simulink model "ihc_lowpass_filter"  (R2020b)
settings: Solver=FixedStepDiscrete  StartTime=0.0  StopTime=stopTime  FixedStep=2.0833333333333333e-05  RelTol=1e-3
values from neighbouring files (symbols this model uses):
  IHCLPcoeffs = [ gainihc*c2LPihc gainihc*c2LPihc 0 1 -c1LPihc 0 ... (first row only)    [ihc_lowpass_filter_parameters.m]
settings Model: Creator=Ross  LastModifiedBy=conno
settings DataIOCC: SaveOutput=off  SaveTime=off  ReturnWorkspaceOutputs=off
settings OptimizationCC: BlockReduction=off  ConditionallyExecuteInputs=off  DefaultParameterBehavior=Inlined
settings DebuggingCC: ReadBeforeWriteMsg=DisableAll  WriteAfterWriteMsg=DisableAll  WriteAfterReadMsg=DisableAll  AlgebraicLoopMsg=error  MultiTaskDSMMsg=none  SingleTaskRateTransMsg=error  PregeneratedLibrarySubsystemCodeDiagnostic=none  ArithmeticOperatorsInVariantConditions=warning
settings HardwareCC: ProdBitPerPointer=32  ProdBitPerSizeT=32  ProdBitPerPtrDiffT=32  ProdLargestAtomicFloat=None  ProdIntDivRoundTo=Undefined  ProdEndianess=Unspecified  ProdWordSize=32  ProdHWDeviceType=ASIC/FPGA->ASIC/FPGA  TargetBitPerPointer=64  TargetBitPerSizeT=64  TargetBitPerPtrDiffT=64  TargetLongLongMode=on  TargetIntDivRoundTo=Zero  TargetEndianess=LittleEndian  TargetWordSize=64  TargetHWDeviceType=Custom Processor->MATLAB Host Computer  ProdEqTarget=off
settings ModelReferenceCC: UpdateModelReferenceTargets=IfOutOfDate
settings SFSimCC: SFSimEcho=off  SimUseLocalCustomCode=off  CustomCodeUndefinedFunction=UseInterfaceOnly
settings RTWCC: RTWUseLocalCustomCode=off

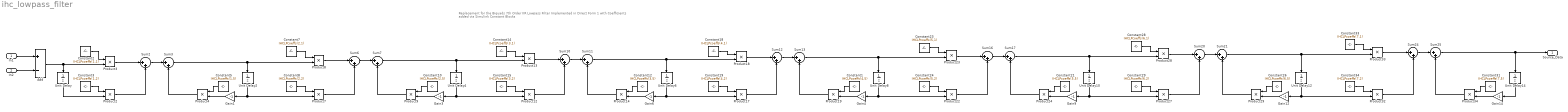
== system ihc_lowpass_filter ==
  note: Replacement for the Biquads
      | 7th Order IIR Lowpass Filter Implemented in Direct Form 1 with Coefficients added via Simulink Constant Blocks
  In1 : Inport  OutDataTypeStr=single  PortDimensions=1  SampleTime=[2.0833333333333333e-05,0]
  In2 : Inport  Port=2  OutDataTypeStr=single  PortDimensions=1  SampleTime=[2.0833333333333333e-05,0]
  Add : Sum  Inputs=+-  RndMeth=Nearest
  Constant1 : Constant  Value=IHCLPcoeffs(4,5)  OutDataTypeStr=single  SampleTime=-1
  Constant10 : Constant  Value=IHCLPcoeffs(2,5)  OutDataTypeStr=single  SampleTime=-1
  Constant12 : Constant  Value=IHCLPcoeffs(3,5)  OutDataTypeStr=single  SampleTime=-1
  Constant14 : Constant  Value=IHCLPcoeffs(3,1)  OutDataTypeStr=single  SampleTime=-1
  Constant15 : Constant  Value=IHCLPcoeffs(3,2)  OutDataTypeStr=single  SampleTime=-1
  Constant18 : Constant  Value=IHCLPcoeffs(4,1)  OutDataTypeStr=single  SampleTime=-1
  Constant19 : Constant  Value=IHCLPcoeffs(4,2)  OutDataTypeStr=single  SampleTime=-1
  Constant2 : Constant  Value=IHCLPcoeffs(1,1)  OutDataTypeStr=single  SampleTime=-1
  Constant21 : Constant  Value=IHCLPcoeffs(5,5)  OutDataTypeStr=single  SampleTime=-1
  Constant23 : Constant  Value=IHCLPcoeffs(5,1)  OutDataTypeStr=single  SampleTime=-1
  Constant24 : Constant  Value=IHCLPcoeffs(5,2)  OutDataTypeStr=single  SampleTime=-1
  Constant26 : Constant  Value=IHCLPcoeffs(6,5)  OutDataTypeStr=single  SampleTime=-1
  Constant28 : Constant  Value=IHCLPcoeffs(6,1)  OutDataTypeStr=single  SampleTime=-1
  Constant29 : Constant  Value=IHCLPcoeffs(6,2)  OutDataTypeStr=single  SampleTime=-1
  Constant3 : Constant  Value=IHCLPcoeffs(1,2)  OutDataTypeStr=single  SampleTime=-1
  Constant31 : Constant  Value=IHCLPcoeffs(7,5)  OutDataTypeStr=single  SampleTime=-1
  Constant33 : Constant  Value=IHCLPcoeffs(7,1)  OutDataTypeStr=single  SampleTime=-1
  Constant34 : Constant  Value=IHCLPcoeffs(7,2)  OutDataTypeStr=single  SampleTime=-1
  Constant5 : Constant  Value=IHCLPcoeffs(1,5)  OutDataTypeStr=single  SampleTime=-1
  Constant7 : Constant  Value=IHCLPcoeffs(2,1)  OutDataTypeStr=single  SampleTime=-1
  Constant8 : Constant  Value=IHCLPcoeffs(2,2)  OutDataTypeStr=single  SampleTime=-1
  Gain{1,3..4,6,9,12,14} (7 alike) : Gain  Gain=-1
  Product{2..4,7..9,12..14,17..19,22..24,27..29,32..34} (21 alike) : Product
  Sum{2..3,6..7,10..13,16..17,20..21,24..25} (14 alike) : Sum  Inputs=|++
  Unit Delay{,2,4,6,8,10,12,14} (8 alike) : UnitDelay  SampleTime=-1  HasFrameUpgradeWarning=on
  Source_Data : Outport  OutDataTypeStr=single  PortDimensions=1  SampleTime=[2.0833333333333333e-05,0]
  wires:
  Constant31/1 -> Product34/1
  Product34/1 -> Sum25/2
  Sum24/1 -> Sum25/1
  Gain14/1 -> Product34/2
  Sum25/1 -> Source_Data/1, Unit Delay14/1
  Product32/1 -> Sum24/2
  Product33/1 -> Sum24/1
  Unit Delay14/1 -> Gain14/1
  Constant34/1 -> Product32/1
  Constant33/1 -> Product33/1
  Constant26/1 -> Product29/1
  Product29/1 -> Sum21/2
  Sum20/1 -> Sum21/1
  Gain12/1 -> Product29/2
  Sum21/1 -> Unit Delay12/1, Product33/2
  Product27/1 -> Sum20/2
  Product28/1 -> Sum20/1
  Unit Delay12/1 -> Product32/2, Gain12/1
  Constant29/1 -> Product27/1
  Constant28/1 -> Product28/1
  Sum12/1 -> Sum13/1
  Constant23/1 -> Product23/1
  Constant2/1 -> Product3/1
  Constant7/1 -> Product8/1
  Add/1 -> Product3/2, Unit Delay/1
  Product8/1 -> Sum6/1
  Constant1/1 -> Product19/1
  Unit Delay4/1 -> Product12/2, Gain3/1
  Product24/1 -> Sum17/2
  Constant24/1 -> Product22/1
  Gain6/1 -> Product14/2
  Sum13/1 -> Unit Delay8/1, Product23/2
  Sum7/1 -> Unit Delay4/1, Product13/2
  Product12/1 -> Sum10/2
  Gain1/1 -> Product4/2
  Product14/1 -> Sum11/2
  Gain4/1 -> Product19/2
  Sum10/1 -> Sum11/1
  Gain9/1 -> Product24/2
  Unit Delay10/1 -> Product27/2, Gain9/1
  Unit Delay6/1 -> Product17/2, Gain6/1
  Product4/1 -> Sum3/2
  Sum11/1 -> Unit Delay6/1, Product18/2
  Product18/1 -> Sum12/1
  Constant15/1 -> Product12/1
  Sum16/1 -> Sum17/1
  Constant19/1 -> Product17/1
  Unit Delay2/1 -> Product7/2, Gain1/1
  Constant21/1 -> Product24/1
  Constant3/1 -> Product2/1
  Product3/1 -> Sum2/1
  Product23/1 -> Sum16/1
  Sum3/1 -> Unit Delay2/1, Product8/2
  Product22/1 -> Sum16/2
  Unit Delay8/1 -> Product22/2, Gain4/1
  Unit Delay/1 -> Product2/2
  Gain3/1 -> Product9/2
  Product17/1 -> Sum12/2
  Product13/1 -> Sum10/1
  Sum17/1 -> Unit Delay10/1, Product28/2
  Constant14/1 -> Product13/1
  Constant12/1 -> Product14/1
  Constant18/1 -> Product18/1
  Product9/1 -> Sum7/2
  Constant5/1 -> Product4/1
  Constant10/1 -> Product9/1
  Product19/1 -> Sum13/2
  Constant8/1 -> Product7/1
  Sum2/1 -> Sum3/1
  Sum6/1 -> Sum7/1
  Product2/1 -> Sum2/2
  Product7/1 -> Sum6/2
  In1/1 -> Add/1
  In2/1 -> Add/2
